simulink model "Quadrotor"  (R2024b)
settings: Solver=VariableStepAuto  StartTime=0.0  StopTime=10.0  RelTol=1e-3
model workspace (MAT data in the model file):
  Ixx = 8.12e-05
  m = 0.506
settings Model: Creator=oscak  LastModifiedBy=oscak

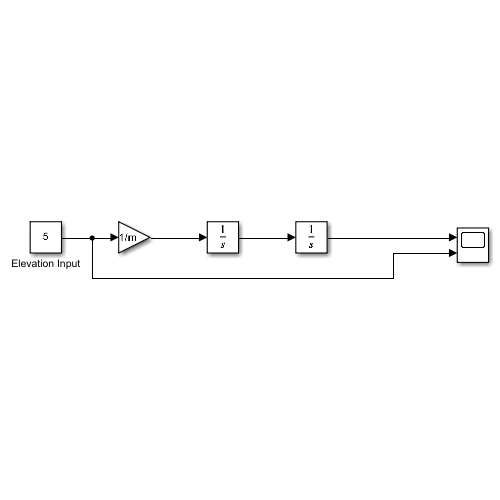
[thumbnail: Simulink's stored preview of the top-level diagram]
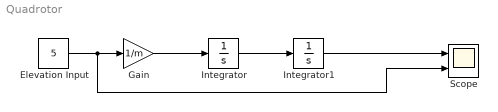
== system Quadrotor ==
  Elevation Input : Constant  Value=5
  Gain : Gain  Gain=1/m
  Integrator : Integrator
  Integrator1 : Integrator
  Scope : Scope  NumInputPorts=2
  wires:
  Elevation Input/1 -> Scope/2, Gain/1
  Gain/1 -> Integrator/1
  Integrator/1 -> Integrator1/1
  Integrator1/1 -> Scope/1
